simulink model "mlf_statemcn"  (R2015b)
settings: Solver=ode45  StartTime=0.0  StopTime=1000  RelTol=1e-3
libraries: simulink x1, hdlsllib x1
settings Model: Creator=amatsumo  LastModifiedBy=amatsumo
settings DataIOCC: SaveFormat=Array
settings DebuggingCC: UnderspecifiedInitializationDetection=Classic  MergeDetectMultiDrivingBlocksExec=none  SolverPrmCheckMsg=warning  StateNameClashWarn=warning
settings HardwareCC: ProdBitPerPointer=32  ProdLargestAtomicFloat=None  ProdIntDivRoundTo=Undefined  ProdEndianess=Unspecified  ProdWordSize=32  ProdHWDeviceType=32-bit Generic
settings GRTTargetCC: GeneratePreprocessorConditionals=Disable all
settings ConfigComp: CovModelRefEnable=Off  CovSFcnEnable=off

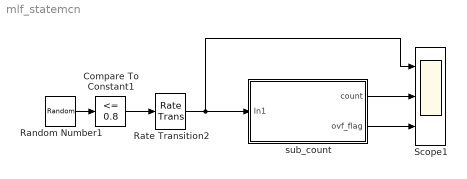
== system mlf_statemcn ==
  Compare To Constant1 : simulink/Logic and Bit Operations/Compare To Constant  relop=<=  const=0.8  OutDataTypeStr=boolean  ZeroCross=off
  Random Number1 : RandomNumber  SampleTime=70
  Rate Transition2 : RateTransition  OutPortSampleTime=1
  Scope1 : Scope  NumInputPorts=3
  sub_count : Subsystem
  wires:
  Random Number1/1 -> Compare To Constant1/1
  Compare To Constant1/1 -> Rate Transition2/1
  Rate Transition2/1 -> sub_count/1(In1), Scope1/1
  sub_count/1(count) -> Scope1/2
  sub_count/2(ovf_flag) -> Scope1/3

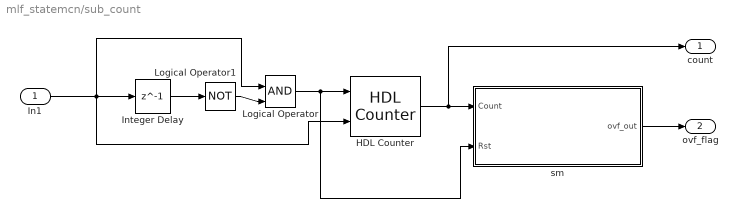
== system mlf_statemcn/sub_count ==
  In1 : Inport
  HDL Counter : hdlsllib/HDL Operations/HDL Counter  CountType=Free running  CountInit=1  CountStep=1  CountMax=100  CountFromType=Initial value  CountFrom=1  CountResetPort=on  CountLoadPort=off  CountEnbPort=on  CountDirPort=off  CountDataType=Unsigned  CountWordLen=8  CountFracLen=0  CountSampTime=1
  Integer Delay : Delay  DelayLength=1  InputProcessing=Inherited
  Logical Operator : Logic  IconShape=distinctive  AllPortsSameDT=off  OutDataTypeStr=boolean
  Logical Operator1 : Logic  Operator=NOT  IconShape=distinctive  AllPortsSameDT=off  OutDataTypeStr=boolean
  sm : MATLAB Function  TreatAsAtomicUnit=on
  count : Outport
  ovf_flag : Outport  Port=2
  wires:
  In1/1 -> Logical Operator/1, HDL Counter/2, Integer Delay/1
  Logical Operator/1 -> sm/2(Rst), HDL Counter/1
  HDL Counter/1 -> sm/1(Count), count/1
  Integer Delay/1 -> Logical Operator1/1
  Logical Operator1/1 -> Logical Operator/2
  sm/1(ovf_out) -> ovf_flag/1

== matlab function mlf_statemcn/sub_count/sm ==
  data: Count input uint8; ovf_out output boolean; Rst input boolean
function ovf_out  = sm(Count, Rst)
%#codegen

persistent state_reg
if isempty(state_reg)
	state_reg = fi(0, 0, 2, 0);
end

Idl = fi(0, 0, 2, 0);
Max = fi(1, 0, 2, 0);
Ovf = fi(2, 0, 2, 0);

switch (state_reg) 
    case Idl,
        if Count >= 255
			state_reg = Max;
			ovf_out = false;
        else
            state_reg = Idl;
			ovf_out = false;
        end
    case Max,
		if Count == 0
            state_reg = Ovf;
			ovf_out = true;
		else
			state_reg = Idl;
			ovf_out = false;
		end
    case Ovf,
		if Rst == 1
			state_reg = Idl;
			ovf_out = false;
		else
			state_reg = Ovf;
			ovf_out = true;
		end
    otherwise,
		ovf_out = false;
end
end
